simulink model "car_model"  (Simulink 7.5)
settings: Solver=ode3  StartTime=0.0  StopTime=4  FixedStep=0.01  RelTol=1e-3
values from neighbouring files (symbols this model uses):
  f_F0 = [0 m*g*l_R*(l_F + l_R)]'    [testCarModel.m]
  f_R0 = [0 m*g*l_R*(l_F + l_R)]'    [testCarModel.m]
  u0 = [f_Fx0, f_Rx0, delta0]'    [testCarModel.m]
  X0 = [Vx0 Vy0 r0 psi0]'    [testCarModel.m]
  Xin0 = [posX0 posY0]'    [testCarModel.m]
settings Model: Creator=oktay  LastModifiedBy=oktay

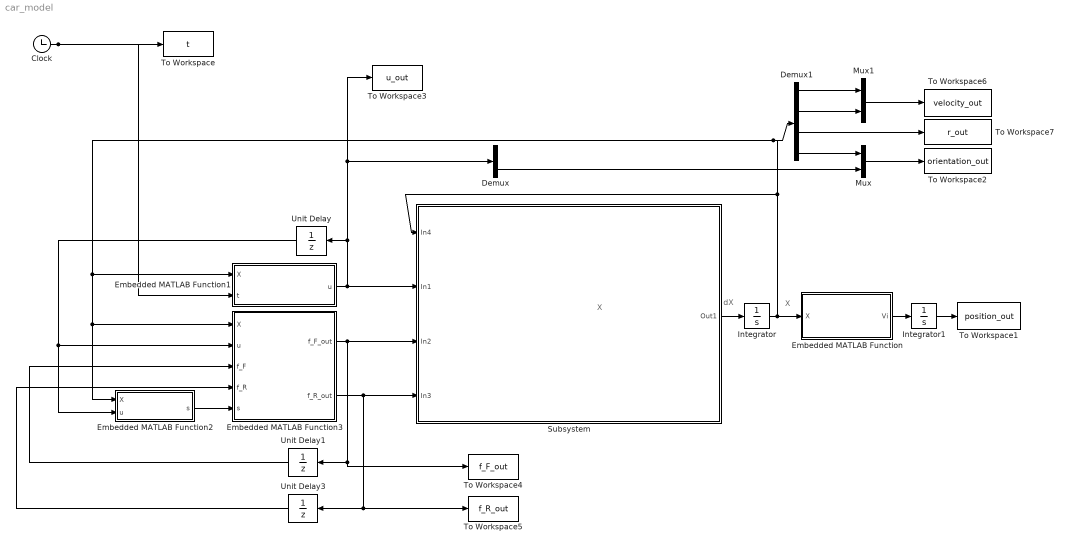
== system car_model ==
  note: X
  note: dX
  note: X
  Clock : Clock
      settings: Decimation=10
  Demux : Demux  Outputs=3
  Demux1 : Demux
  Embedded MATLAB Function : Stateflow chart  TreatAsAtomicUnit=on
  Embedded MATLAB Function1 : Stateflow chart  TreatAsAtomicUnit=on
  Embedded MATLAB Function2 : Stateflow chart  TreatAsAtomicUnit=on
  Embedded MATLAB Function3 : Stateflow chart  TreatAsAtomicUnit=on
  Integrator : Integrator  InitialCondition=X0
  Integrator1 : Integrator  InitialCondition=Xin0
  Mux : Mux  Inputs=2
  Mux1 : Mux  Inputs=2
  Subsystem : Subsystem
      mask Display: image(imread('car_logo.png'))
  To Workspace : ToWorkspace  VariableName=t  SampleTime=-1  SaveFormat=Array
  To Workspace1 : ToWorkspace  VariableName=position_out  SampleTime=-1  SaveFormat=Array
  To Workspace2 : ToWorkspace  VariableName=orientation_out  SampleTime=-1  SaveFormat=Array
  To Workspace3 : ToWorkspace  VariableName=u_out  SampleTime=-1  SaveFormat=Array
  To Workspace4 : ToWorkspace  VariableName=f_F_out  SampleTime=-1  SaveFormat=Array
  To Workspace5 : ToWorkspace  VariableName=f_R_out  SampleTime=-1  SaveFormat=Array
  To Workspace6 : ToWorkspace  VariableName=velocity_out  SampleTime=-1  SaveFormat=Array
  To Workspace7 : ToWorkspace  VariableName=r_out  SampleTime=-1  SaveFormat=Array
  Unit Delay : UnitDelay  X0=u0  SampleTime=-1
  Unit Delay1 : UnitDelay  X0=f_F0  SampleTime=-1
  Unit Delay3 : UnitDelay  X0=f_R0  SampleTime=0
  wires:
  Subsystem/1(Out1) -> Integrator/1
  Embedded MATLAB Function3/1(f_F_out) -> Subsystem/3(In2), Unit Delay1/1, To Workspace4/1
  Embedded MATLAB Function3/2(f_R_out) -> Subsystem/4(In3), Unit Delay3/1, To Workspace5/1
  Embedded MATLAB Function1/1(u) -> Subsystem/2(In1), Unit Delay/1, Demux/1, To Workspace3/1
  Embedded MATLAB Function2/1(s) -> Embedded MATLAB Function3/5(s)
  Unit Delay/1 -> Embedded MATLAB Function2/2(u), Embedded MATLAB Function3/2(u)
  Unit Delay1/1 -> Embedded MATLAB Function3/3(f_F)
  Unit Delay3/1 -> Embedded MATLAB Function3/4(f_R)
  Integrator/1 -> Embedded MATLAB Function/1(X), Embedded MATLAB Function1/1(X), Embedded MATLAB Function3/1(X), Embedded MATLAB Function2/1(X), Demux1/1, Subsystem/1(In4)
  Embedded MATLAB Function/1(Vi) -> Integrator1/1
  Integrator1/1 -> To Workspace1/1
  Clock/1 -> To Workspace/1, Embedded MATLAB Function1/2(t)
  Demux1/4 -> Mux/1
  Demux/3 -> Mux/2
  Mux/1 -> To Workspace2/1
  Demux1/1 -> Mux1/1
  Demux1/2 -> Mux1/2
  Mux1/1 -> To Workspace6/1
  Demux1/3 -> To Workspace7/1

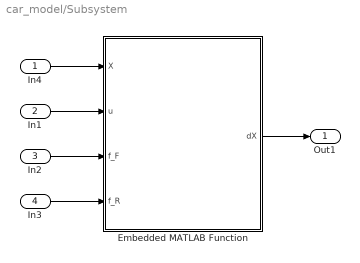
== system car_model/Subsystem ==
  In4 : Inport
  In1 : Inport  Port=2
  In2 : Inport  Port=3
  In3 : Inport  Port=4
  Embedded MATLAB Function : Stateflow chart  TreatAsAtomicUnit=on
  Out1 : Outport
  wires:
  In1/1 -> Embedded MATLAB Function/2(u)
  In2/1 -> Embedded MATLAB Function/3(f_F)
  In3/1 -> Embedded MATLAB Function/4(f_R)
  Embedded MATLAB Function/1(dX) -> Out1/1
  In4/1 -> Embedded MATLAB Function/1(X)

== matlab function Embedded MATLAB Function1 ==
  data: u output double; X input double; t input double
function u = controller(X,t)
%#eml
global CONSTANTS

f_Fx = 0;
f_Rx = CONSTANTS.f_Rx_max;

delta = -45/180*pi;
% if (t > .36)
%    delta = -45*pi/180;
% else
    
%    delta = 45*pi/180;
% end

u = [f_Fx; f_Rx; delta];

== matlab function Subsystem/Embedded MATLAB Function ==
  data: X input double; u input double; f_F input double; f_R input double; dX output double
function dX = car_dynamics(X, u, f_F, f_R)
%#eml

% m = param.m;
% Iz = param.Iz;
% l_F = param.l_F;
% l_R = param.l_R;
% B = param.B;
% C = param.C;
% mu = param.mu;
% delta_max = param.delta_max;

m = 1450;
Iz = 2740;
l_F = 1.1;
l_R = 1.6;

Vx = X(1);
Vy = X(2);
r = X(3);
psi = X(4);

f_Fx  = u(1);
f_Rx  = u(2);
delta = u(3);

f_Fy = f_F(1);
f_Fz = f_F(2);

f_Ry = f_R(1);
f_Rz = f_R(2);


dVx = 1/m*(f_Fx*cos(delta) - f_Fy*sin(delta) + f_Rx) + Vy*r;
dVy = 1/m*(f_Fx*sin(delta) + f_Fy*cos(delta) + f_Ry) - Vx*r;
dr = 1/Iz*((f_Fy*cos(delta) + f_Fx*sin(delta))*l_F - f_Ry*l_R);
dpsi = r; 

dX = [dVx dVy dr dpsi]';

== matlab function Embedded MATLAB Function2 ==
  data: X input double; s output double; u input double
function s = lateral_slips( X, u)
%#eml

    % l_F = param.l_F;
    % l_R = param.l_R;

    l_F = 1.1;
    l_R = 1.6;

    Vx  = X(1);
    Vy  = X(2);
    r   = X(3);
    psi = X(4); 

    f_Fx  = u(1);
    f_Rx  = u(2);
    delta = u(3);


    if (Vx == 0 && Vy ==0)
        beta = 0;
    else
        beta = atan(Vy/Vx);
    end

    V = sqrt(Vx^2 + Vy^2);

    s_Fy_num = (V*sin(beta-delta) + r*l_F*cos(delta));
    s_Fy_denum = (V*cos(beta-delta) + r*l_F*sin(delta));

    if (s_Fy_num == 0 && s_Fy_denum == 0)
        s_Fy = 0;
    else
        s_Fy = s_Fy_num/s_Fy_denum;
    end

    s_Ry_num = (V*sin(beta) - r*l_R);
    s_Ry_denum = (V*cos(beta));

    if (s_Ry_num == 0 && s_Ry_denum == 0)
        s_Ry = 0;
    else
        s_Ry = s_Ry_num/s_Ry_denum;
    end

    s = [s_Fy; s_Ry];

end

== matlab function Embedded MATLAB Function3 ==
  data: f_F_out output double; f_R_out output double; X input double; u input double; f_F input double; f_R input double; s input double
function [f_F_out, f_R_out] = forces (X, u, f_F, f_R, s)

% m = param.m;
% l_F = param.l_F;
% l_R = param.l_R;
% mu = param.mu;

global CONSTANTS

m = 1450;
l_F = 1.1;
l_R = 1.6;
mu = 0.5;
C = 1.4;
B = 7;

g = 9.82;


Vx  = X(1); 
Vy  = X(2);
r   = X(3);
psi = X(4);

f_Fx  = u(1);
f_Rx  = u(2);
delta = u(3);

f_Fy = f_F(1);  
f_Fz = f_F(2);

f_Ry = f_R(1);  
f_Rz = f_R(2);

s_Fy = s(1);
s_Ry = s(2); 


f_Fz_out = m*g*l_R*(l_F + l_R);
f_Rz_out = m*g*l_F*(l_F + l_R);

f_Fy_max = sqrt((mu*f_Fz)^2 - f_Fx^2);
f_Ry_max = sqrt((mu*f_Rz)^2 - f_Rx^2);

f_Fy_out = -f_Fy_max*sin(C*atan(B*s_Fy)); 
f_Ry_out = -f_Ry_max*sin(C*atan(B*s_Ry));

f_F_out = [f_Fy_out; f_Fz_out];
f_R_out = [f_Ry_out; f_Rz_out];

== matlab function Embedded MATLAB Function ==
  data: X input double; Vi output double
function Vi = Body2Inertia(X)
%#eml

Vx = X(1);
Vy = X(2);
r = X(3);
psi = X(4);

T = [cos(psi) -sin(psi); sin(psi) cos(psi)]; 

Vi = T*[Vx; Vy];
